simulink model "sim_6"  (R2022b)
settings: Solver=FixedStepAuto  StartTime=0.0  StopTime=100  FixedStep=0.05  RelTol=1e-3
values from neighbouring files (symbols this model uses):
  K = 1.0121    [gen_pid.m]    (also in getFitness.m = [Pop(i,1)]; identa.m; params.m)
  T = 0.891    [gen_pid.m]    (also in getFitness.m = [Pop(i,2) 1]; identa.m; params.m)
  Td = 0.2811    [gen_pid.m]    (also in getFitness.m = Pop(i,3); identa.m; params.m)
settings Model: Creator=DFUNDO  LastModifiedBy=DFUNDO

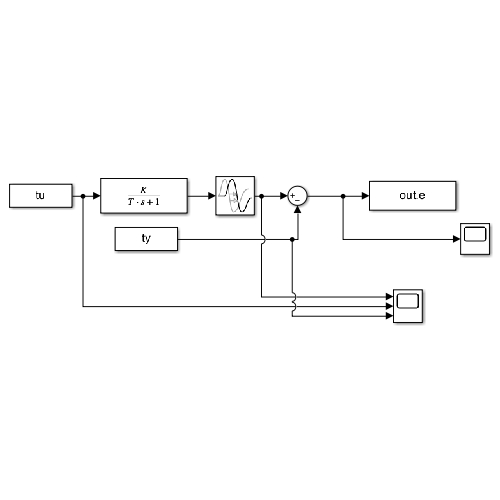
[thumbnail: Simulink's stored preview of the top-level diagram]
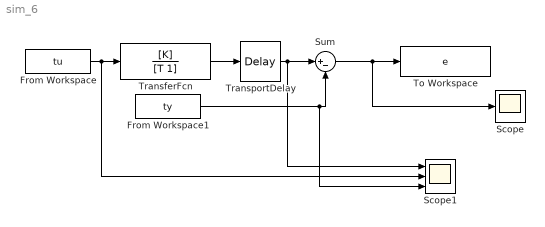
== system sim_6 ==
  From Workspace : FromWorkspace  VariableName=tu
  From Workspace1 : FromWorkspace  VariableName=ty
  Scope : Scope
  Scope1 : Scope  NumInputPorts=3
  Sum : Sum  Inputs=|+-
  To Workspace : ToWorkspace  VariableName=e  SampleTime=-1
      settings: Save2DSignal=2-D array (concatenate along first dimension)
  TransferFcn : TransferFcn  Numerator=[K]  Denominator=[T 1]
  TransportDelay : TransportDelay  DelayTime=Td
  wires:
  From Workspace/1 -> Scope1/2, TransferFcn/1
  TransportDelay/1 -> Scope1/1, Sum/1
  From Workspace1/1 -> Scope1/3, Sum/2
  Sum/1 -> Scope/1, To Workspace/1
  TransferFcn/1 -> TransportDelay/1
